simulink model "guidanceOrbitExample"  (R2020b)
settings: Solver=FixedStepAuto  StartTime=0.0  StopTime=inf  FixedStep=0.01  RelTol=1e-3
libraries: pid_lib x1, ksplib x1
settings Model: DataDictionary=kspdemo.sldd  EnablePacing=on  PacingRate=2  Creator=brianhannan  LastModifiedBy=bhannan

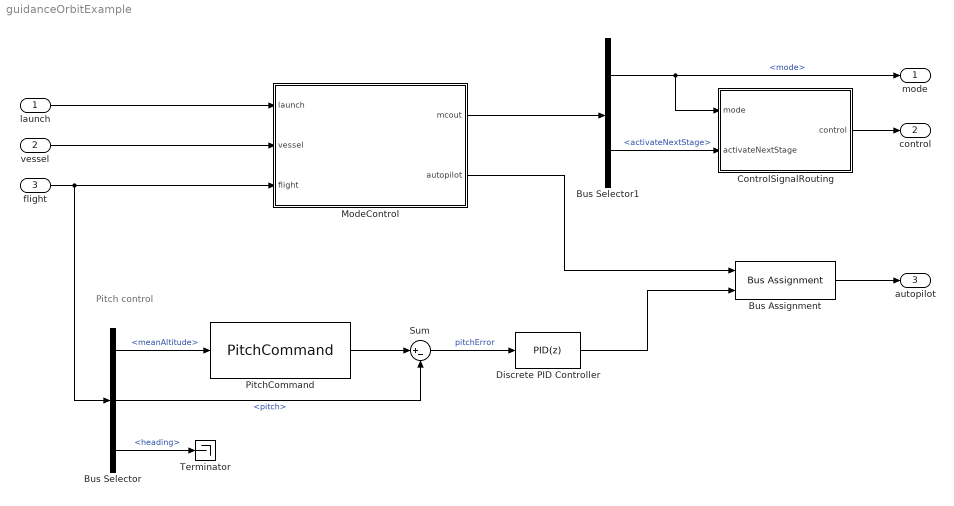
== system guidanceOrbitExample ==
  note: Pitch control
  launch : Inport  OutDataTypeStr=boolean  PortDimensions=1
  vessel : Inport  Port=2  OutDataTypeStr=Bus: vesselRx
  flight : Inport  Port=3  OutDataTypeStr=Bus: flight
  Bus Assignment : BusAssignment  AssignedSignals=targetPitch
  Bus Selector : BusSelector  OutputSignals=meanAltitude,pitch,heading
  Bus Selector1 : BusSelector  OutputSignals=mode,activateNextStage
  ControlSignalRouting : Subsystem
  Discrete PID Controller : pid_lib/PID Controller  Controller=PID  Form=Parallel  TimeDomain=Discrete-time  UseExternalTs=off  SampleTime=-1  IntegratorMethod=Forward Euler  FilterMethod=Forward Euler  ControllerParametersSource=internal  P=2  I=1  D=0  UseFilter=on  N=100  TunerSelectOption=Transfer Function Based (PID Tuner App)  InitialConditionSource=internal  InitialConditionForIntegrator=0  InitialConditionForFilter=0  DifferentiatorICPrevScaledInput=0  ExternalReset=none  TrackingMode=off  Kt=1  LimitOutput=on  SatLimitsSource=internal  UpperSaturationLimit=90  LowerSaturationLimit=-90  LinearizeAsGain=off  AntiWindupMode=none  Kb=1  POutMin=[]  POutMax=[]  IOutMin=[]  IOutMax=[]  DOutMin=[]  DOutMax=[]  NOutMin=[]  NOutMax=[]  SumOutMin=[]  SumOutMax=[]  SaturationOutMin=[]  SaturationOutMax=[]  PParamMin=[]  PParamMax=[]  IParamMin=[]  IParamMax=[]  DParamMin=[]  DParamMax=[]  NParamMin=[]  NParamMax=[]  KbParamMin=[]  KbParamMax=[]  KtParamMin=[]  KtParamMax=[]  KbOutMin=[]  KbOutMax=[]  KtOutMin=[]  KtOutMax=[]  IntegratorOutMin=[]  IntegratorOutMax=[]  FilterOutMin=[]  FilterOutMax=[]  SumI1OutMin=[]  SumI1OutMax=[]  SumI2OutMin=[]  SumI2OutMax=[]  SumI3OutMin=[]  SumI3OutMax=[]  SumI4OutMin=[]  SumI4OutMax=[]  SumDOutMin=[]  SumDOutMax=[]  DifferentiatorOutMin=[]  DifferentiatorOutMax=[]  FilterDiffOutCoefMin=[]  FilterDiffOutCoefMax=[]  ReciprocalOutMin=[]  ReciprocalOutMax=[]  SumDenOutMin=[]  SumDenOutMax=[]  SumNumOutMin=[]  SumNumOutMax=[]  DivideOutMin=[]  DivideOutMax=[]  UdiffTsProdOutMin=[]  UdiffTsProdOutMax=[]  NTsProdOutMin=[]  NTsProdOutMax=[]  UintegralTsProdOutMin=[]  UintegralTsProdOutMax=[]  UngainTsProdOutMin=[]  UngainTsProdOutMax=[]  IntegratorContinuousStateAttributes=''  IntegratorStateMustResolveToSignalObject=off  IntegratorRTWStateStorageClass=Auto  FilterContinuousStateAttributes=''  FilterStateMustResolveToSignalObject=off  FilterRTWStateStorageClass=Auto  ParallelPVariant=InternalParameters  IdealPVariant=Disabled  IVariant=InternalParameters  DVariant=InternalParameters  IntegratorVariant=Discrete  SatVariant=Enabled  AWVariant=Passthrough  PCopyVariant=Disabled  TRVariant=Disabled  FdbkBlocksVariant=Forward  IdealPFdbkVariant=Disabled  SatFdbkVariant=Disabled  DerivativeFilterVariant=ForwardEulerFilter  NVariant=InternalParameters  NCopyVariant=Disabled  FilterICVariant=InternalICsFilter  IntegratorICVariant=InternalICs  ExternalResetVariant=Disabled  TRSumVariant=Passthrough  SumFdbkVariant=Disabled  SumVariant=Sum_PID  TsampFilterVariant=InternalTs  TsampNgainVariant=Passthrough  TsampIntegralVariant=Passthrough  ExternalSaturationOutDataTypeStr=Inherit: Same as second input
  ModeControl : Subsystem  mask(FlightMode){}
      mask help: Flight mode state machine. Performs high-level mission logic (launch, staging, etc.).
      mask Display:
      | disp('Flight Mode')
      | 
      | port_label('input',1,'launch')
      | port_label('input',2,'vessel')
      | port_label('input',3,'flight')
      | 
      | port_label('output',1,'control')
      | port_label('output',2,'autopilot')
  PitchCommand : ksplib/PitchCommand  altitudeVals=[1000, 10000, 30000, 40000]  pitchVals=[0, 5, 15, 20]
  Sum : Sum  Inputs=|+-
  Terminator : Terminator
  mode : Outport
  control : Outport  Port=2  OutDataTypeStr=Bus: control
  autopilot : Outport  Port=3  OutDataTypeStr=Bus: autopilot
  wires:
  launch/1 -> ModeControl/1(launch)
  ModeControl/2(autopilot) -> Bus Assignment/1
  vessel/1 -> ModeControl/2(vessel)
  flight/1 -> Bus Selector/1, ModeControl/3(flight)
  Bus Selector/3 -> Terminator/1  "<heading>"
  Sum/1 -> Discrete PID Controller/1  "pitchError"
  ModeControl/1(mcout) -> Bus Selector1/1
  Bus Assignment/1 -> autopilot/1
  Discrete PID Controller/1 -> Bus Assignment/2
  Bus Selector/1 -> PitchCommand/1  "<meanAltitude>"
  Bus Selector/2 -> Sum/2  "<pitch>"
  PitchCommand/1 -> Sum/1
  Bus Selector1/2 -> ControlSignalRouting/2(activateNextStage)  "<activateNextStage>"
  ControlSignalRouting/1(control) -> control/1
  Bus Selector1/1 -> ControlSignalRouting/1(mode), mode/1  "<mode>"

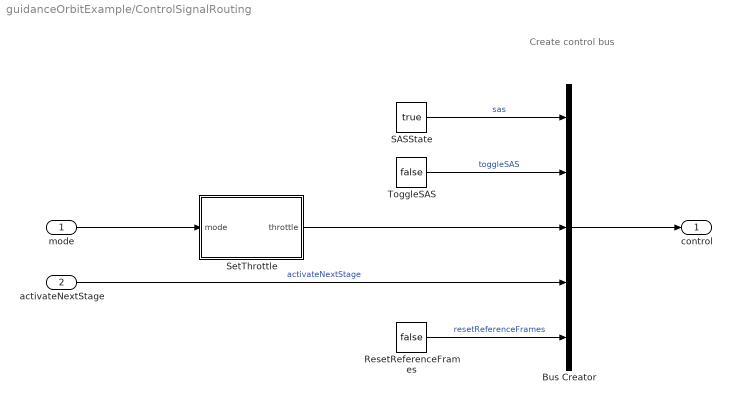
== system guidanceOrbitExample/ControlSignalRouting ==
  note: Create control bus
  mode : Inport
  activateNextStage : Inport  Port=2
  Bus Creator : BusCreator  Inputs=5  OutDataTypeStr=Bus: control  NonVirtualBus=on
      settings: InheritFromInputs=off
  ResetReferenceFrames : Constant  Value=false  OutDataTypeStr=boolean
  SASState : Constant  Value=true  OutDataTypeStr=boolean
  SetThrottle : Subsystem
  ToggleSAS : Constant  Value=false  OutDataTypeStr=boolean
  control : Outport  OutDataTypeStr=Bus: control
  wires:
  Bus Creator/1 -> control/1
  SASState/1 -> Bus Creator/1  "sas"
  ResetReferenceFrames/1 -> Bus Creator/5  "resetReferenceFrames"
  ToggleSAS/1 -> Bus Creator/2  "toggleSAS"
  activateNextStage/1 -> Bus Creator/4  "activateNextStage"
  SetThrottle/1(throttle) -> Bus Creator/3
  mode/1 -> SetThrottle/1(mode)

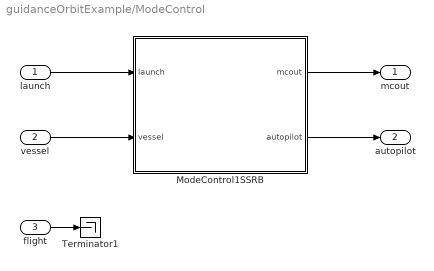
== system guidanceOrbitExample/ModeControl ==
  launch : Inport
  vessel : Inport  Port=2
  flight : Inport  Port=3
  ModeControl1SSRB : Stateflow chart  TreatAsAtomicUnit=on
  Terminator1 : Terminator
  mcout : Outport
  autopilot : Outport  Port=2
  wires:
  flight/1 -> Terminator1/1
  vessel/1 -> ModeControl1SSRB/2(vessel)
  ModeControl1SSRB/1(mcout) -> mcout/1
  launch/1 -> ModeControl1SSRB/1(launch)
  ModeControl1SSRB/2(autopilot) -> autopilot/1

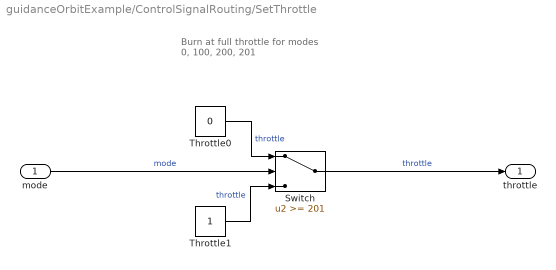
== system guidanceOrbitExample/ControlSignalRouting/SetThrottle ==
  note: Burn at full throttle for modes 0, 100, 200, 201
  mode : Inport
  Switch : Switch  Threshold=201
  Throttle0 : Constant  Value=0  OutDataTypeStr=double
  Throttle1 : Constant  OutDataTypeStr=double
  throttle : Outport  OutMin=0  OutMax=1  OutDataTypeStr=double
  wires:
  mode/1 -> Switch/2  "mode"
  Switch/1 -> throttle/1  "throttle"
  Throttle1/1 -> Switch/3  "throttle"
  Throttle0/1 -> Switch/1  "throttle"

== stateflow chart guidanceOrbitExample/ModeControl/ModeControl1SSRB ==
  note: Guidance moding logic for a two-stage liquid fuel rocket.
  note: Stage 1 separation is triggered when stage 1 liquid fuel is spent.
  note: Stage separation
  note: Stage 2 burn
  state Prelaunch
    en:
    mcout.mode = int16(-100);
    autopilot.targetPitch = 90;
    autopilot.targetHeading = 90;
    autopilot.engage = true;
  state Launch
    en:
    mcout.mode = int16(0);
    state PreFlightChecks
      en:
      % to do: add prelaunch check logic
      launchChecksOK = true;
    (default) -> PreFlightChecks
  state Stage1
    en:
    mcout.mode = int16(100);
    du:
    if ~launchCmdSent
    mcout.activateNextStage = true;
    launchCmdSent = true;
    else
    mcout.activateNextStage = false;
    end
  state Stage1Separation
    en:
    mcout.mode = int16(200);
    du:
    if ~stage1sepCmdSent
    mcout.activateNextStage = true;
    stage1sepCmdSent = true;
    else
    mcout.activateNextStage = false;
    end
  state Stage2
    en:
    mcout.mode = int16(201);
    du:
    if ~stage2ignitionCmdSent
    mcout.activateNextStage = true;
    stage2ignitionCmdSent = true;
    else
    mcout.activateNextStage = false;
    end
  state MECO
    en:
    mcout.mode = int16(202);
    du:
    % do nothing
  (default) -> Prelaunch
  Prelaunch -> Launch : [launch == true]
  Stage1 -> Stage1Separation : [vessel.liquidFuelAmt < 180.1]
  Launch -> (junction 31) [order 1] : [launchChecksOK == true]
  (junction 31) -> Stage1 : [after(1.0,sec)]
  Stage1Separation -> Stage2 : [after(0.5,sec)]
  Launch -> Prelaunch [order 2] : [launchChecksOK == false]
  Stage2 -> MECO : [vessel.apoapsisAltitude > 70e3]
  data: launch input boolean size=1; mcout output Bus: mcout size=1; launchChecksOK local boolean =true; autopilot output Bus: autopilot; stage1sepCmdSent local boolean =false; launchCmdSent local boolean =false; vessel input; stage2ignitionCmdSent local boolean =false
